simulink model "CM020A_Bmw5441McuCfg"  (R2013b)
settings: Solver=FixedStepDiscrete  SolverMode=SingleTasking  StartTime=0.0  StopTime=1  FixedStep=0.0005  RelTol=1e-3
PreLoadFcn:
  | CM020A_Bmw5441McuCfg_DataDict
values from neighbouring files (symbols this model uses):
  ADC0CFGANDUSE_ADCD0SGVCEP2_CNT_U08 = DataDict.Constant    [CM020A_Bmw5441McuCfg_DataDict.m]
  ADC0CFGANDUSE_ADCD0SGVCEP3_CNT_U08 = DataDict.Constant    [CM020A_Bmw5441McuCfg_DataDict.m]
  ADC0CFGANDUSE_ADCD0SGVCSP2_CNT_U08 = DataDict.Constant    [CM020A_Bmw5441McuCfg_DataDict.m]
  ADC0CFGANDUSE_ADCD0SGVCSP3_CNT_U08 = DataDict.Constant    [CM020A_Bmw5441McuCfg_DataDict.m]
  ADC0CFGANDUSE_ADCD0VCR00_CNT_U32 = DataDict.Constant    [CM020A_Bmw5441McuCfg_DataDict.m]
  ADC0CFGANDUSE_ADCD0VCR01_CNT_U32 = DataDict.Constant    [CM020A_Bmw5441McuCfg_DataDict.m]
  ADC0CFGANDUSE_ADCD0VCR02_CNT_U32 = DataDict.Constant    [CM020A_Bmw5441McuCfg_DataDict.m]
  ADC0CFGANDUSE_ADCD0VCR03_CNT_U32 = DataDict.Constant    [CM020A_Bmw5441McuCfg_DataDict.m]
  ADC0CFGANDUSE_ADCD0VCR04_CNT_U32 = DataDict.Constant    [CM020A_Bmw5441McuCfg_DataDict.m]
  ADC0CFGANDUSE_ADCD0VCR05_CNT_U32 = DataDict.Constant    [CM020A_Bmw5441McuCfg_DataDict.m]
  ADC0CFGANDUSE_ADCD0VCR06_CNT_U32 = DataDict.Constant    [CM020A_Bmw5441McuCfg_DataDict.m]
  ADC0CFGANDUSE_ADCD0VCR07_CNT_U32 = DataDict.Constant    [CM020A_Bmw5441McuCfg_DataDict.m]
  ADC0CFGANDUSE_ADCD0VCR08_CNT_U32 = DataDict.Constant    [CM020A_Bmw5441McuCfg_DataDict.m]
  ADC0CFGANDUSE_ADCD0VCR09_CNT_U32 = DataDict.Constant    [CM020A_Bmw5441McuCfg_DataDict.m]
  ADC0CFGANDUSE_ADCD0VCR10_CNT_U32 = DataDict.Constant    [CM020A_Bmw5441McuCfg_DataDict.m]
  ADC0CFGANDUSE_ADCD0VCR11_CNT_U32 = DataDict.Constant    [CM020A_Bmw5441McuCfg_DataDict.m]
  ADC0CFGANDUSE_ADCD0VCR12_CNT_U32 = DataDict.Constant    [CM020A_Bmw5441McuCfg_DataDict.m]
  ADC0CFGANDUSE_ADCD0VCR13_CNT_U32 = DataDict.Constant    [CM020A_Bmw5441McuCfg_DataDict.m]
  ADC0CFGANDUSE_ADCD0VCR14_CNT_U32 = DataDict.Constant    [CM020A_Bmw5441McuCfg_DataDict.m]
  ADC0CFGANDUSE_ADCD0VCR15_CNT_U32 = DataDict.Constant    [CM020A_Bmw5441McuCfg_DataDict.m]
  ADC0CFGANDUSE_ADCD0VCR16_CNT_U32 = DataDict.Constant    [CM020A_Bmw5441McuCfg_DataDict.m]
  ADC0CFGANDUSE_ADCD0VCR17_CNT_U32 = DataDict.Constant    [CM020A_Bmw5441McuCfg_DataDict.m]
  ADC0CFGANDUSE_ADCD0VCR18_CNT_U32 = DataDict.Constant    [CM020A_Bmw5441McuCfg_DataDict.m]
  ADC0CFGANDUSE_ADCD0VCR19_CNT_U32 = DataDict.Constant    [CM020A_Bmw5441McuCfg_DataDict.m]
  ADC0CFGANDUSE_ADCD0VCR20_CNT_U32 = DataDict.Constant    [CM020A_Bmw5441McuCfg_DataDict.m]
  ADC0CFGANDUSE_ADCSCAGFAC_VOLTPERCNT_F32 = DataDict.Constant    [CM020A_Bmw5441McuCfg_DataDict.m]
  ADC1CFGANDUSE_ADCD1SGVCEP2_CNT_U08 = DataDict.Constant    [CM020A_Bmw5441McuCfg_DataDict.m]
  ADC1CFGANDUSE_ADCD1SGVCEP3_CNT_U08 = DataDict.Constant    [CM020A_Bmw5441McuCfg_DataDict.m]
  ADC1CFGANDUSE_ADCD1SGVCSP2_CNT_U08 = DataDict.Constant    [CM020A_Bmw5441McuCfg_DataDict.m]
  ADC1CFGANDUSE_ADCD1SGVCSP3_CNT_U08 = DataDict.Constant    [CM020A_Bmw5441McuCfg_DataDict.m]
  ADC1CFGANDUSE_ADCD1VCR00_CNT_U32 = DataDict.Constant    [CM020A_Bmw5441McuCfg_DataDict.m]
  ADC1CFGANDUSE_ADCD1VCR01_CNT_U32 = DataDict.Constant    [CM020A_Bmw5441McuCfg_DataDict.m]
  ADC1CFGANDUSE_ADCD1VCR02_CNT_U32 = DataDict.Constant    [CM020A_Bmw5441McuCfg_DataDict.m]
  ADC1CFGANDUSE_ADCD1VCR03_CNT_U32 = DataDict.Constant    [CM020A_Bmw5441McuCfg_DataDict.m]
  ADC1CFGANDUSE_ADCD1VCR04_CNT_U32 = DataDict.Constant    [CM020A_Bmw5441McuCfg_DataDict.m]
  ADC1CFGANDUSE_ADCD1VCR05_CNT_U32 = DataDict.Constant    [CM020A_Bmw5441McuCfg_DataDict.m]
  ADC1CFGANDUSE_ADCD1VCR06_CNT_U32 = DataDict.Constant    [CM020A_Bmw5441McuCfg_DataDict.m]
  ADC1CFGANDUSE_ADCD1VCR07_CNT_U32 = DataDict.Constant    [CM020A_Bmw5441McuCfg_DataDict.m]
  ADC1CFGANDUSE_ADCD1VCR08_CNT_U32 = DataDict.Constant    [CM020A_Bmw5441McuCfg_DataDict.m]
  ADC1CFGANDUSE_ADCD1VCR09_CNT_U32 = DataDict.Constant    [CM020A_Bmw5441McuCfg_DataDict.m]
  ADC1CFGANDUSE_ADCD1VCR10_CNT_U32 = DataDict.Constant    [CM020A_Bmw5441McuCfg_DataDict.m]
  ADC1CFGANDUSE_ADCD1VCR11_CNT_U32 = DataDict.Constant    [CM020A_Bmw5441McuCfg_DataDict.m]
  ADC1CFGANDUSE_ADCD1VCR12_CNT_U32 = DataDict.Constant    [CM020A_Bmw5441McuCfg_DataDict.m]
  ADC1CFGANDUSE_ADCD1VCR13_CNT_U32 = DataDict.Constant    [CM020A_Bmw5441McuCfg_DataDict.m]
  ADC1CFGANDUSE_ADCD1VCR14_CNT_U32 = DataDict.Constant    [CM020A_Bmw5441McuCfg_DataDict.m]
  ADC1CFGANDUSE_ADCD1VCR15_CNT_U32 = DataDict.Constant    [CM020A_Bmw5441McuCfg_DataDict.m]
  ADC1CFGANDUSE_ADCD1VCR16_CNT_U32 = DataDict.Constant    [CM020A_Bmw5441McuCfg_DataDict.m]
  ADC1CFGANDUSE_ADCD1VCR17_CNT_U32 = DataDict.Constant    [CM020A_Bmw5441McuCfg_DataDict.m]
  ADC1CFGANDUSE_ADCD1VCR18_CNT_U32 = DataDict.Constant    [CM020A_Bmw5441McuCfg_DataDict.m]
  ADC1CFGANDUSE_ADCD1VCR19_CNT_U32 = DataDict.Constant    [CM020A_Bmw5441McuCfg_DataDict.m]
  ADC1CFGANDUSE_ADCD1VCR20_CNT_U32 = DataDict.Constant    [CM020A_Bmw5441McuCfg_DataDict.m]
  ADCDIAGC_DYNDIAGFAILSTEP_CNT_U16 = DataDict.Constant    [CM020A_Bmw5441McuCfg_DataDict.m]
  ADCDIAGC_DYNDIAGPASSSTEP_CNT_U16 = DataDict.Constant    [CM020A_Bmw5441McuCfg_DataDict.m]
  BATTRTNCURR_CURRESTIMDIFTHD_AMPR_F32 = DataDict.Constant    [CM020A_Bmw5441McuCfg_DataDict.m]
  BATTRTNCURR_FAILSTEP_CNT_U16 = DataDict.Constant    [CM020A_Bmw5441McuCfg_DataDict.m]
  BATTRTNCURR_FASTLOOPPROC_CNT_LOGL = DataDict.Constant    [CM020A_Bmw5441McuCfg_DataDict.m]
  BATTRTNCURR_FILCUTFREQ_HZ_F32 = DataDict.Constant    [CM020A_Bmw5441McuCfg_DataDict.m]
  BATTRTNCURR_GAIN_AMPRPERVOLT_F32 = DataDict.Constant    [CM020A_Bmw5441McuCfg_DataDict.m]
  BATTRTNCURR_LOWRTHD_AMPR_F32 = DataDict.Constant    [CM020A_Bmw5441McuCfg_DataDict.m]
  BATTRTNCURR_OFFSET_VOLT_F32 = DataDict.Constant    [CM020A_Bmw5441McuCfg_DataDict.m]
  BATTRTNCURR_OUTPMAX_AMPR_F32 = DataDict.Constant    [CM020A_Bmw5441McuCfg_DataDict.m]
  BATTRTNCURR_OUTPMIN_AMPR_F32 = DataDict.Constant    [CM020A_Bmw5441McuCfg_DataDict.m]
  BATTRTNCURR_PASSSTEP_CNT_U16 = DataDict.Constant    [CM020A_Bmw5441McuCfg_DataDict.m]
  BATTRTNCURR_UPPRTHD_AMPR_F32 = DataDict.Constant    [CM020A_Bmw5441McuCfg_DataDict.m]
  BATTVLTGSCAGFAC_ULS_F32 = DataDict.Constant    [CM020A_Bmw5441McuCfg_DataDict.m]
  BATTVLTGSWD1SCAGFAC_ULS_F32 = DataDict.Constant    [CM020A_Bmw5441McuCfg_DataDict.m]
  ECUTMEAS_DFTT_DEGCGRD_F32 = DataDict.Constant    [CM020A_Bmw5441McuCfg_DataDict.m]
  ECUTMEAS_ECUTX_VOLT_U3P13 = DataDict.Constant    [CM020A_Bmw5441McuCfg_DataDict.m]
  ECUTMEAS_ECUTY_DEGCGRD_S8P7 = DataDict.Constant    [CM020A_Bmw5441McuCfg_DataDict.m]
  ECUTMEAS_FILTAU_HZ_F32 = DataDict.Constant    [CM020A_Bmw5441McuCfg_DataDict.m]
  ECUTMEAS_NTC0X045FAILSTEP_CNT_U16 = DataDict.Constant    [CM020A_Bmw5441McuCfg_DataDict.m]
  ECUTMEAS_NTC0X045PASSSTEP_CNT_U16 = DataDict.Constant    [CM020A_Bmw5441McuCfg_DataDict.m]
  ECUTMEAS_RNGDIAGCMAX_DEGCGRD_F32 = DataDict.Constant    [CM020A_Bmw5441McuCfg_DataDict.m]
  ECUTMEAS_RNGDIAGCMIN_DEGCGRD_F32 = DataDict.Constant    [CM020A_Bmw5441McuCfg_DataDict.m]
  ELECGLBPRM_IVTRCNT_CNT_U08 = DataDict.Constant    [CM020A_Bmw5441McuCfg_DataDict.m]
  ELECGLBPRM_PWMFRQMAX_HZ_U32 = DataDict.Constant    [CM020A_Bmw5441McuCfg_DataDict.m]
  ELECGLBPRM_PWMFRQMIN_HZ_U32 = DataDict.Constant    [CM020A_Bmw5441McuCfg_DataDict.m]
  ELECGLBPRM_PWMPERDMAX_NANOSEC_U32 = DataDict.Constant    [CM020A_Bmw5441McuCfg_DataDict.m]
  ELECGLBPRM_PWMPERDMIN_NANOSEC_U32 = DataDict.Constant    [CM020A_Bmw5441McuCfg_DataDict.m]
  ELECGLBPRM_PWMPERDNOM_MICROSEC_U7P9 = DataDict.Constant    [CM020A_Bmw5441McuCfg_DataDict.m]
  ELECGLBPRM_PWMPERDNOMX2_SEC_F32 = DataDict.Constant    [CM020A_Bmw5441McuCfg_DataDict.m]
  FLTINJENA = DataDict.Constant    [CM020A_Bmw5441McuCfg_DataDict.m]
  HWTQ4MEAS_HWTQ4RNGCHKPRTCLNTCNR_CNT_ENUM = DataDict.Constant    [CM020A_Bmw5441McuCfg_DataDict.m]
  HWTQ4MEAS_HWTQ4SCANOTPRFMMFGNTCNR_CNT_ENUM = DataDict.Constant    [CM020A_Bmw5441McuCfg_DataDict.m]
  HWTQ4MEAS_HWTQ4TRIMNOTPRFMMFGNTCNR_CNT_ENUM = DataDict.Constant    [CM020A_Bmw5441McuCfg_DataDict.m]
  HWTQ4MEAS_HWTQBARSTFN_NMPDEG_F32 = DataDict.Constant    [CM020A_Bmw5441McuCfg_DataDict.m]
  HWTQ4MEAS_HWTQOFFS_VOLT_F32 = DataDict.Constant    [CM020A_Bmw5441McuCfg_DataDict.m]
  HWTQ4MEAS_HWTQSNSRSCANOMVAL_VOLTPDEG_F32 = DataDict.Constant    [CM020A_Bmw5441McuCfg_DataDict.m]
  HWTQ5MEAS_HWTQ5RNGCHKPRTCLNTCNR_CNT_ENUM = DataDict.Constant    [CM020A_Bmw5441McuCfg_DataDict.m]
  HWTQ5MEAS_HWTQ5SCANOTPRFMMFGNTCNR_CNT_ENUM = DataDict.Constant    [CM020A_Bmw5441McuCfg_DataDict.m]
  HWTQ5MEAS_HWTQ5TRIMNOTPRFMMFGNTCNR_CNT_ENUM = DataDict.Constant    [CM020A_Bmw5441McuCfg_DataDict.m]
  HWTQ5MEAS_HWTQBARSTFN_NMPDEG_F32 = DataDict.Constant    [CM020A_Bmw5441McuCfg_DataDict.m]
  HWTQ5MEAS_HWTQOFFS_VOLT_F32 = DataDict.Constant    [CM020A_Bmw5441McuCfg_DataDict.m]
  HWTQ5MEAS_HWTQSNSRSCANOMVAL_VOLTPDEG_F32 = DataDict.Constant    [CM020A_Bmw5441McuCfg_DataDict.m]
  MOTAG0MEAS_MOTAG0PRTCLFLTNTCNR_CNT_ENUM = DataDict.Constant    [CM020A_Bmw5441McuCfg_DataDict.m]
  MOTAG1MEAS_MOTAG1PRTCLFLTNTCNR_CNT_ENUM = DataDict.Constant    [CM020A_Bmw5441McuCfg_DataDict.m]
  MOTAG3MEAS_SNSRRLVBITWIDTHEXP_CNT_U08 = DataDict.Constant    [CM020A_Bmw5441McuCfg_DataDict.m]
  MOTAG4MEAS_SNSRRLVBITWIDTHEXP_CNT_U08 = DataDict.Constant    [CM020A_Bmw5441McuCfg_DataDict.m]
  RVSBATTPROTN_FAILSTEP_CNT_U16 = DataDict.Constant    [CM020A_Bmw5441McuCfg_DataDict.m]
  RVSBATTPROTN_GNDMEASDVLTGHILIMN_VOLT_F32 = DataDict.Constant    [CM020A_Bmw5441McuCfg_DataDict.m]
  RVSBATTPROTN_GNDMEASDVLTGLOLIMN_VOLT_F32 = DataDict.Constant    [CM020A_Bmw5441McuCfg_DataDict.m]
  RVSBATTPROTN_PASSSTEP_CNT_U16 = DataDict.Constant    [CM020A_Bmw5441McuCfg_DataDict.m]
  RVSBATTPROTN_RTNMEASDVLTGHILIMN_VOLT_F32 = DataDict.Constant    [CM020A_Bmw5441McuCfg_DataDict.m]
  RVSBATTPROTN_RTNMEASDVLTGLOLIMN_VOLT_F32 = DataDict.Constant    [CM020A_Bmw5441McuCfg_DataDict.m]
  RVSBATTPROTN_RVSFLTTHD_VOLT_F32 = DataDict.Constant    [CM020A_Bmw5441McuCfg_DataDict.m]
  SWPENA = DataDict.Constant    [CM020A_Bmw5441McuCfg_DataDict.m]
  TUNSELNAUTHY_XCPVEHSPDTHD_KPH_F32 = DataDict.Constant    [CM020A_Bmw5441McuCfg_DataDict.m]
libraries: CM020A_Bmw5441McuCfg_ModelLibrary x82, simulink x24
(part 3 of 3)

== system CM020A_Bmw5441McuCfg/Bmw5441McuCfg/Bmw5441McuCfgPer3/OtherSignals ==
  Constant : Constant  Value=true  OutDataTypeStr=boolean
  CopyRight2 : Subsystem  Description=|  mask(Copyright Information){none=on}
      | Copyright info block.                                               
      |                                                                     
      | Place copyright information at the top of every subsystem in design.
      mask prompts: none "No parameters"
      mask help: Place copyright information at the top of every subsystem in design.
      mask Display:
      | NxtrConf = 'Nexteer Confidential';
      | 
      | sys = bdroot; %handle for the current model ("system")
      | first = get_param(sys,'Created');
      | first = first(end-3:end);  %year is last four digits
      | 
      | last = get_param(sys,'LastModifiedDate');
      | if isempty(last)
      |     last = datestr(now,'yyyy');
      | else
      |     last = last(end-3:end);
      | end
      | 
      | if strcmp(first,last)
      |     fprintf('%s -- Copyright %s Nexteer',NxtrConf,first)
      | else
      |     fprintf('%s -- %s%s- %s Nexteer',NxtrConf,char(169),first,last)
      | end
  MotDrvr1IninTestCmpl : Outport
  wires:
  Constant/1 -> MotDrvr1IninTestCmpl/1

== system CM020A_Bmw5441McuCfg/Bmw5441McuCfg/Bmw5441McuCfgInit1/Do Not Code/CopyRight2 ==

== system CM020A_Bmw5441McuCfg/Bmw5441McuCfg/Bmw5441McuCfgInit1/Register Initialization/CopyRight2 ==

== system CM020A_Bmw5441McuCfg/Bmw5441McuCfg/Bmw5441McuCfgInit2/Process Initial Adc0/CopyRight2 ==

== system CM020A_Bmw5441McuCfg/Bmw5441McuCfg/Bmw5441McuCfgInit2/Wait for ADC Conversion to Complete/CopyRight2 ==

== system CM020A_Bmw5441McuCfg/Bmw5441McuCfg/Bmw5441McuCfgInit2/Wait for ADC Conversion to Complete/GetRefTmr1MicroSec32bit ==
  CopyRight2 : Subsystem  Description=|  mask(Copyright Information){none=on}
      | Copyright info block.                                               
      |                                                                     
      | Place copyright information at the top of every subsystem in design.
      mask prompts: none "No parameters"
      mask help: Place copyright information at the top of every subsystem in design.
      mask Display:
      | NxtrConf = 'Nexteer Confidential';
      | 
      | sys = bdroot; %handle for the current model ("system")
      | first = get_param(sys,'Created');
      | if(isempty(first))
      |     first = datestr(now,'yyyy');
      | else
      |     first = first(end-3:end);  %year is last four digits
      | end
      | 
      | last = get_param(sys,'LastModifiedDate');
      | if isempty(last)
      |     last = datestr(now,'yyyy');
      | else
      |     last = last(end-3:end);
      | end
      | 
      | if strcmp(first,last)
      |     fprintf('%s -- Copyright %s Nexteer',NxtrConf,first)
      | else
      |     fprintf('%s -- %s%s- %s Nexteer',NxtrConf,char(169),first,last)
      | end
  Ground : Ground
  RefTmr : Outport
  wires:
  Ground/1 -> RefTmr/1

== system CM020A_Bmw5441McuCfg/Bmw5441McuCfg/Bmw5441McuCfgInit2/Wait for ADC Conversion to Complete/GetTiSpan1MicroSec32bit ==
  RefTmr : Inport
  CopyRight2 : Subsystem  Description=|  mask(Copyright Information){none=on}
      | Copyright info block.                                               
      |                                                                     
      | Place copyright information at the top of every subsystem in design.
      mask prompts: none "No parameters"
      mask help: Place copyright information at the top of every subsystem in design.
      mask Display:
      | NxtrConf = 'Nexteer Confidential';
      | 
      | sys = bdroot; %handle for the current model ("system")
      | first = get_param(sys,'Created');
      | if(isempty(first))
      |     first = datestr(now,'yyyy');
      | else
      |     first = first(end-3:end);  %year is last four digits
      | end
      | 
      | last = get_param(sys,'LastModifiedDate');
      | if isempty(last)
      |     last = datestr(now,'yyyy');
      | else
      |     last = last(end-3:end);
      | end
      | 
      | if strcmp(first,last)
      |     fprintf('%s -- Copyright %s Nexteer',NxtrConf,first)
      | else
      |     fprintf('%s -- %s%s- %s Nexteer',NxtrConf,char(169),first,last)
      | end
  Ground : Ground
  Terminator : Terminator
  TiSpan : Outport
  wires:
  Ground/1 -> TiSpan/1
  RefTmr/1 -> Terminator/1

== system CM020A_Bmw5441McuCfg/Bmw5441McuCfg/Bmw5441McuCfgInit3/Process Initial Adc1/CopyRight2 ==

== system CM020A_Bmw5441McuCfg/Bmw5441McuCfg/Bmw5441McuCfgPer3/Adc0Faild Processing/CopyRight2 ==

== system CM020A_Bmw5441McuCfg/Bmw5441McuCfg/Bmw5441McuCfgPer3/Adc1Faild Processing/CopyRight2 ==

== system CM020A_Bmw5441McuCfg/Bmw5441McuCfg/Bmw5441McuCfgPer3/OtherSignals/CopyRight2 ==

== system CM020A_Bmw5441McuCfg/Bmw5441McuCfg/Bmw5441McuCfgInit2/Wait for ADC Conversion to Complete/GetRefTmr1MicroSec32bit/CopyRight2 ==

== system CM020A_Bmw5441McuCfg/Bmw5441McuCfg/Bmw5441McuCfgInit2/Wait for ADC Conversion to Complete/GetTiSpan1MicroSec32bit/CopyRight2 ==
